simulink model "boundingbox"  (R2018a)
settings: Solver=VariableStepAuto  StartTime=0.0  StopTime=10.0  RelTol=1e-3
libraries: simulink x127
(part 3 of 4)

== system boundingbox/generate_proximity_sensor_readings/Subsystem1/distance_to_bounding_box/calculate_intersection 2 ==
  note: for two 2d vectors U=(Ux,Uy) V=(Vx,Vy)the crossproduct isU x V = Ux*Vy-Uy*Vx
  vertex_1 : Inport
  vertex_2 : Inport  Port=2
  "origin " : Inport  Port=3
  ray : Inport  Port=4
  AND : Logic  Inputs=3  IconShape=distinctive  AllPortsSameDT=off  OutDataTypeStr=boolean
  Abs : Abs
  Compare To Constant : simulink/Logic and Bit Operations/Compare To Constant  relop=<=  const=1  OutDataTypeStr=boolean
  Compare To Zero : simulink/Logic and Bit Operations/Compare To Zero  relop=>=  OutDataTypeStr=boolean
  Compare To Zero1 : simulink/Logic and Bit Operations/Compare To Zero  relop=>=  OutDataTypeStr=boolean
  Demux{,1..6} (7 alike) : Demux  Outputs=2
  Divide : Product  Inputs=*/
  Divide1 : Product  Inputs=*/
  Dot Product : DotProduct  InputSameDT=on  OutDataTypeStr=Inherit: Inherit via internal rule
  Dot Product1 : DotProduct  InputSameDT=on  OutDataTypeStr=Inherit: Inherit via internal rule
  Dot Product2 : DotProduct  InputSameDT=on  OutDataTypeStr=Inherit: Inherit via internal rule
  Gain : Gain  Gain=-1
  Multiply : Product
  Multiply1 : Product
  Subtract{,1,3..4} (4 alike) : Sum  Inputs=-+
  Subtract2 : Sum  Inputs=+-
  Vector Concatenate : Concatenate
  Vector Concatenate1 : Concatenate
  Vector Concatenate2 : Concatenate
  distance : Outport
  intersection (0,1) : Outport  Port=2
  wires:
  Compare To Constant/1 -> AND/3
  Compare To Zero/1 -> AND/2
  Divide1/1 -> Compare To Zero/1, Compare To Constant/1
  AND/1 -> intersection (0,1)/1
  Dot Product2/1 -> Divide1/2
  Dot Product1/1 -> Divide1/1
  Multiply1/1 -> Subtract2/2
  Multiply/1 -> Subtract2/1
  Demux2/1 -> Multiply1/2
  Demux1/2 -> Multiply1/1
  Demux2/2 -> Multiply/2
  Demux1/1 -> Multiply/1
  Abs/1 -> Divide/1
  Subtract2/1 -> Abs/1
  Dot Product/1 -> Divide/2
  Divide/1 -> Compare To Zero1/1, distance/1
  Subtract/1 -> Vector Concatenate1/2
  Vector Concatenate/1 -> Dot Product/2, Dot Product1/2, Dot Product2/2
  Demux/1 -> Vector Concatenate/2
  Gain/1 -> Vector Concatenate/1
  Demux/2 -> Gain/1
  ray/1 -> Demux/1
  vertex_2/1 -> Demux3/1
  vertex_1/1 -> Demux6/1, Demux4/1
  "origin "/1 -> Demux5/1
  Demux5/1 -> Subtract3/2
  Demux6/1 -> Subtract3/1
  Demux6/2 -> Subtract/1
  Demux5/2 -> Subtract/2
  Demux4/1 -> Subtract1/1
  Demux4/2 -> Subtract4/1
  Demux3/1 -> Subtract1/2
  Demux3/2 -> Subtract4/2
  Subtract3/1 -> Vector Concatenate1/1
  Vector Concatenate1/1 -> Dot Product1/1, Demux1/1
  Subtract4/1 -> Vector Concatenate2/2
  Subtract1/1 -> Vector Concatenate2/1
  Vector Concatenate2/1 -> Dot Product/1, Demux2/1, Dot Product2/1
  Compare To Zero1/1 -> AND/1

== system boundingbox/generate_proximity_sensor_readings/Subsystem1/distance_to_bounding_box/calculate_intersection 3 ==
  note: for two 2d vectors U=(Ux,Uy) V=(Vx,Vy)the crossproduct isU x V = Ux*Vy-Uy*Vx
  vertex_1 : Inport
  vertex_2 : Inport  Port=2
  "origin " : Inport  Port=3
  ray : Inport  Port=4
  AND : Logic  Inputs=3  IconShape=distinctive  AllPortsSameDT=off  OutDataTypeStr=boolean
  Abs : Abs
  Compare To Constant : simulink/Logic and Bit Operations/Compare To Constant  relop=<=  const=1  OutDataTypeStr=boolean
  Compare To Zero : simulink/Logic and Bit Operations/Compare To Zero  relop=>=  OutDataTypeStr=boolean
  Compare To Zero1 : simulink/Logic and Bit Operations/Compare To Zero  relop=>=  OutDataTypeStr=boolean
  Demux{,1..6} (7 alike) : Demux  Outputs=2
  Divide : Product  Inputs=*/
  Divide1 : Product  Inputs=*/
  Dot Product : DotProduct  InputSameDT=on  OutDataTypeStr=Inherit: Inherit via internal rule
  Dot Product1 : DotProduct  InputSameDT=on  OutDataTypeStr=Inherit: Inherit via internal rule
  Dot Product2 : DotProduct  InputSameDT=on  OutDataTypeStr=Inherit: Inherit via internal rule
  Gain : Gain  Gain=-1
  Multiply : Product
  Multiply1 : Product
  Subtract{,1,3..4} (4 alike) : Sum  Inputs=-+
  Subtract2 : Sum  Inputs=+-
  Vector Concatenate : Concatenate
  Vector Concatenate1 : Concatenate
  Vector Concatenate2 : Concatenate
  distance : Outport
  intersection (0,1) : Outport  Port=2
  wires:
  Compare To Zero1/1 -> AND/1
  Vector Concatenate2/1 -> Dot Product2/1, Demux2/1, Dot Product/1
  Subtract1/1 -> Vector Concatenate2/1
  Subtract4/1 -> Vector Concatenate2/2
  Vector Concatenate1/1 -> Demux1/1, Dot Product1/1
  Subtract3/1 -> Vector Concatenate1/1
  Demux3/2 -> Subtract4/2
  Demux3/1 -> Subtract1/2
  Demux4/2 -> Subtract4/1
  Demux4/1 -> Subtract1/1
  Demux5/2 -> Subtract/2
  Demux6/2 -> Subtract/1
  Demux6/1 -> Subtract3/1
  Demux5/1 -> Subtract3/2
  "origin "/1 -> Demux5/1
  vertex_1/1 -> Demux4/1, Demux6/1
  vertex_2/1 -> Demux3/1
  ray/1 -> Demux/1
  Demux/2 -> Gain/1
  Gain/1 -> Vector Concatenate/1
  Demux/1 -> Vector Concatenate/2
  Vector Concatenate/1 -> Dot Product2/2, Dot Product1/2, Dot Product/2
  Subtract/1 -> Vector Concatenate1/2
  Divide/1 -> distance/1, Compare To Zero1/1
  Dot Product/1 -> Divide/2
  Subtract2/1 -> Abs/1
  Abs/1 -> Divide/1
  Demux1/1 -> Multiply/1
  Demux2/2 -> Multiply/2
  Demux1/2 -> Multiply1/1
  Demux2/1 -> Multiply1/2
  Multiply/1 -> Subtract2/1
  Multiply1/1 -> Subtract2/2
  Dot Product1/1 -> Divide1/1
  Dot Product2/1 -> Divide1/2
  AND/1 -> intersection (0,1)/1
  Divide1/1 -> Compare To Constant/1, Compare To Zero/1
  Compare To Zero/1 -> AND/2
  Compare To Constant/1 -> AND/3

== system boundingbox/generate_proximity_sensor_readings/Subsystem1/distance_to_bounding_box1/calculate_intersection  ==
  note: for two 2d vectors U=(Ux,Uy) V=(Vx,Vy)the crossproduct isU x V = Ux*Vy-Uy*Vx
  vertex_1 : Inport
  vertex_2 : Inport  Port=2
  "origin " : Inport  Port=3
  ray : Inport  Port=4
  AND : Logic  Inputs=3  IconShape=distinctive  AllPortsSameDT=off  OutDataTypeStr=boolean
  Abs : Abs
  Compare To Constant : simulink/Logic and Bit Operations/Compare To Constant  relop=<=  const=1  OutDataTypeStr=boolean
  Compare To Zero : simulink/Logic and Bit Operations/Compare To Zero  relop=>=  OutDataTypeStr=boolean
  Compare To Zero1 : simulink/Logic and Bit Operations/Compare To Zero  relop=>=  OutDataTypeStr=boolean
  Demux{,1..6} (7 alike) : Demux  Outputs=2
  Divide : Product  Inputs=*/
  Divide1 : Product  Inputs=*/
  Dot Product : DotProduct  InputSameDT=on  OutDataTypeStr=Inherit: Inherit via internal rule
  Dot Product1 : DotProduct  InputSameDT=on  OutDataTypeStr=Inherit: Inherit via internal rule
  Dot Product2 : DotProduct  InputSameDT=on  OutDataTypeStr=Inherit: Inherit via internal rule
  Gain : Gain  Gain=-1
  Multiply : Product
  Multiply1 : Product
  Subtract{,1,3..4} (4 alike) : Sum  Inputs=-+
  Subtract2 : Sum  Inputs=+-
  Vector Concatenate : Concatenate
  Vector Concatenate1 : Concatenate
  Vector Concatenate2 : Concatenate
  distance : Outport
  intersection (0,1) : Outport  Port=2
  wires:
  Compare To Constant/1 -> AND/3
  Compare To Zero/1 -> AND/2
  Divide1/1 -> Compare To Zero/1, Compare To Constant/1
  AND/1 -> intersection (0,1)/1
  Dot Product2/1 -> Divide1/2
  Dot Product1/1 -> Divide1/1
  Multiply1/1 -> Subtract2/2
  Multiply/1 -> Subtract2/1
  Demux2/1 -> Multiply1/2
  Demux1/2 -> Multiply1/1
  Demux2/2 -> Multiply/2
  Demux1/1 -> Multiply/1
  Abs/1 -> Divide/1
  Subtract2/1 -> Abs/1
  Dot Product/1 -> Divide/2
  Divide/1 -> Compare To Zero1/1, distance/1
  Subtract/1 -> Vector Concatenate1/2
  Vector Concatenate/1 -> Dot Product/2, Dot Product1/2, Dot Product2/2
  Demux/1 -> Vector Concatenate/2
  Gain/1 -> Vector Concatenate/1
  Demux/2 -> Gain/1
  ray/1 -> Demux/1
  vertex_2/1 -> Demux3/1
  vertex_1/1 -> Demux6/1, Demux4/1
  "origin "/1 -> Demux5/1
  Demux5/1 -> Subtract3/2
  Demux6/1 -> Subtract3/1
  Demux6/2 -> Subtract/1
  Demux5/2 -> Subtract/2
  Demux4/1 -> Subtract1/1
  Demux4/2 -> Subtract4/1
  Demux3/1 -> Subtract1/2
  Demux3/2 -> Subtract4/2
  Subtract3/1 -> Vector Concatenate1/1
  Vector Concatenate1/1 -> Dot Product1/1, Demux1/1
  Subtract4/1 -> Vector Concatenate2/2
  Subtract1/1 -> Vector Concatenate2/1
  Vector Concatenate2/1 -> Dot Product/1, Demux2/1, Dot Product2/1
  Compare To Zero1/1 -> AND/1

== system boundingbox/generate_proximity_sensor_readings/Subsystem1/distance_to_bounding_box1/calculate_intersection 1 ==
  note: for two 2d vectors U=(Ux,Uy) V=(Vx,Vy)the crossproduct isU x V = Ux*Vy-Uy*Vx
  vertex_1 : Inport
  vertex_2 : Inport  Port=2
  "origin " : Inport  Port=3
  ray : Inport  Port=4
  AND : Logic  Inputs=3  IconShape=distinctive  AllPortsSameDT=off  OutDataTypeStr=boolean
  Abs : Abs
  Compare To Constant : simulink/Logic and Bit Operations/Compare To Constant  relop=<=  const=1  OutDataTypeStr=boolean
  Compare To Zero : simulink/Logic and Bit Operations/Compare To Zero  relop=>=  OutDataTypeStr=boolean
  Compare To Zero1 : simulink/Logic and Bit Operations/Compare To Zero  relop=>=  OutDataTypeStr=boolean
  Demux{,1..6} (7 alike) : Demux  Outputs=2
  Divide : Product  Inputs=*/
  Divide1 : Product  Inputs=*/
  Dot Product : DotProduct  InputSameDT=on  OutDataTypeStr=Inherit: Inherit via internal rule
  Dot Product1 : DotProduct  InputSameDT=on  OutDataTypeStr=Inherit: Inherit via internal rule
  Dot Product2 : DotProduct  InputSameDT=on  OutDataTypeStr=Inherit: Inherit via internal rule
  Gain : Gain  Gain=-1
  Multiply : Product
  Multiply1 : Product
  Subtract{,1,3..4} (4 alike) : Sum  Inputs=-+
  Subtract2 : Sum  Inputs=+-
  Vector Concatenate : Concatenate
  Vector Concatenate1 : Concatenate
  Vector Concatenate2 : Concatenate
  distance : Outport
  intersection (0,1) : Outport  Port=2
  wires:
  Compare To Zero1/1 -> AND/1
  Vector Concatenate2/1 -> Dot Product2/1, Demux2/1, Dot Product/1
  Subtract1/1 -> Vector Concatenate2/1
  Subtract4/1 -> Vector Concatenate2/2
  Vector Concatenate1/1 -> Demux1/1, Dot Product1/1
  Subtract3/1 -> Vector Concatenate1/1
  Demux3/2 -> Subtract4/2
  Demux3/1 -> Subtract1/2
  Demux4/2 -> Subtract4/1
  Demux4/1 -> Subtract1/1
  Demux5/2 -> Subtract/2
  Demux6/2 -> Subtract/1
  Demux6/1 -> Subtract3/1
  Demux5/1 -> Subtract3/2
  "origin "/1 -> Demux5/1
  vertex_1/1 -> Demux4/1, Demux6/1
  vertex_2/1 -> Demux3/1
  ray/1 -> Demux/1
  Demux/2 -> Gain/1
  Gain/1 -> Vector Concatenate/1
  Demux/1 -> Vector Concatenate/2
  Vector Concatenate/1 -> Dot Product2/2, Dot Product1/2, Dot Product/2
  Subtract/1 -> Vector Concatenate1/2
  Divide/1 -> distance/1, Compare To Zero1/1
  Dot Product/1 -> Divide/2
  Subtract2/1 -> Abs/1
  Abs/1 -> Divide/1
  Demux1/1 -> Multiply/1
  Demux2/2 -> Multiply/2
  Demux1/2 -> Multiply1/1
  Demux2/1 -> Multiply1/2
  Multiply/1 -> Subtract2/1
  Multiply1/1 -> Subtract2/2
  Dot Product1/1 -> Divide1/1
  Dot Product2/1 -> Divide1/2
  AND/1 -> intersection (0,1)/1
  Divide1/1 -> Compare To Constant/1, Compare To Zero/1
  Compare To Zero/1 -> AND/2
  Compare To Constant/1 -> AND/3

== system boundingbox/generate_proximity_sensor_readings/Subsystem1/distance_to_bounding_box1/calculate_intersection 2 ==
  note: for two 2d vectors U=(Ux,Uy) V=(Vx,Vy)the crossproduct isU x V = Ux*Vy-Uy*Vx
  vertex_1 : Inport
  vertex_2 : Inport  Port=2
  "origin " : Inport  Port=3
  ray : Inport  Port=4
  AND : Logic  Inputs=3  IconShape=distinctive  AllPortsSameDT=off  OutDataTypeStr=boolean
  Abs : Abs
  Compare To Constant : simulink/Logic and Bit Operations/Compare To Constant  relop=<=  const=1  OutDataTypeStr=boolean
  Compare To Zero : simulink/Logic and Bit Operations/Compare To Zero  relop=>=  OutDataTypeStr=boolean
  Compare To Zero1 : simulink/Logic and Bit Operations/Compare To Zero  relop=>=  OutDataTypeStr=boolean
  Demux{,1..6} (7 alike) : Demux  Outputs=2
  Divide : Product  Inputs=*/
  Divide1 : Product  Inputs=*/
  Dot Product : DotProduct  InputSameDT=on  OutDataTypeStr=Inherit: Inherit via internal rule
  Dot Product1 : DotProduct  InputSameDT=on  OutDataTypeStr=Inherit: Inherit via internal rule
  Dot Product2 : DotProduct  InputSameDT=on  OutDataTypeStr=Inherit: Inherit via internal rule
  Gain : Gain  Gain=-1
  Multiply : Product
  Multiply1 : Product
  Subtract{,1,3..4} (4 alike) : Sum  Inputs=-+
  Subtract2 : Sum  Inputs=+-
  Vector Concatenate : Concatenate
  Vector Concatenate1 : Concatenate
  Vector Concatenate2 : Concatenate
  distance : Outport
  intersection (0,1) : Outport  Port=2
  wires:
  Compare To Constant/1 -> AND/3
  Compare To Zero/1 -> AND/2
  Divide1/1 -> Compare To Zero/1, Compare To Constant/1
  AND/1 -> intersection (0,1)/1
  Dot Product2/1 -> Divide1/2
  Dot Product1/1 -> Divide1/1
  Multiply1/1 -> Subtract2/2
  Multiply/1 -> Subtract2/1
  Demux2/1 -> Multiply1/2
  Demux1/2 -> Multiply1/1
  Demux2/2 -> Multiply/2
  Demux1/1 -> Multiply/1
  Abs/1 -> Divide/1
  Subtract2/1 -> Abs/1
  Dot Product/1 -> Divide/2
  Divide/1 -> Compare To Zero1/1, distance/1
  Subtract/1 -> Vector Concatenate1/2
  Vector Concatenate/1 -> Dot Product/2, Dot Product1/2, Dot Product2/2
  Demux/1 -> Vector Concatenate/2
  Gain/1 -> Vector Concatenate/1
  Demux/2 -> Gain/1
  ray/1 -> Demux/1
  vertex_2/1 -> Demux3/1
  vertex_1/1 -> Demux6/1, Demux4/1
  "origin "/1 -> Demux5/1
  Demux5/1 -> Subtract3/2
  Demux6/1 -> Subtract3/1
  Demux6/2 -> Subtract/1
  Demux5/2 -> Subtract/2
  Demux4/1 -> Subtract1/1
  Demux4/2 -> Subtract4/1
  Demux3/1 -> Subtract1/2
  Demux3/2 -> Subtract4/2
  Subtract3/1 -> Vector Concatenate1/1
  Vector Concatenate1/1 -> Dot Product1/1, Demux1/1
  Subtract4/1 -> Vector Concatenate2/2
  Subtract1/1 -> Vector Concatenate2/1
  Vector Concatenate2/1 -> Dot Product/1, Demux2/1, Dot Product2/1
  Compare To Zero1/1 -> AND/1

== system boundingbox/generate_proximity_sensor_readings/Subsystem1/distance_to_bounding_box1/calculate_intersection 3 ==
  note: for two 2d vectors U=(Ux,Uy) V=(Vx,Vy)the crossproduct isU x V = Ux*Vy-Uy*Vx
  vertex_1 : Inport
  vertex_2 : Inport  Port=2
  "origin " : Inport  Port=3
  ray : Inport  Port=4
  AND : Logic  Inputs=3  IconShape=distinctive  AllPortsSameDT=off  OutDataTypeStr=boolean
  Abs : Abs
  Compare To Constant : simulink/Logic and Bit Operations/Compare To Constant  relop=<=  const=1  OutDataTypeStr=boolean
  Compare To Zero : simulink/Logic and Bit Operations/Compare To Zero  relop=>=  OutDataTypeStr=boolean
  Compare To Zero1 : simulink/Logic and Bit Operations/Compare To Zero  relop=>=  OutDataTypeStr=boolean
  Demux{,1..6} (7 alike) : Demux  Outputs=2
  Divide : Product  Inputs=*/
  Divide1 : Product  Inputs=*/
  Dot Product : DotProduct  InputSameDT=on  OutDataTypeStr=Inherit: Inherit via internal rule
  Dot Product1 : DotProduct  InputSameDT=on  OutDataTypeStr=Inherit: Inherit via internal rule
  Dot Product2 : DotProduct  InputSameDT=on  OutDataTypeStr=Inherit: Inherit via internal rule
  Gain : Gain  Gain=-1
  Multiply : Product
  Multiply1 : Product
  Subtract{,1,3..4} (4 alike) : Sum  Inputs=-+
  Subtract2 : Sum  Inputs=+-
  Vector Concatenate : Concatenate
  Vector Concatenate1 : Concatenate
  Vector Concatenate2 : Concatenate
  distance : Outport
  intersection (0,1) : Outport  Port=2
  wires:
  Compare To Zero1/1 -> AND/1
  Vector Concatenate2/1 -> Dot Product2/1, Demux2/1, Dot Product/1
  Subtract1/1 -> Vector Concatenate2/1
  Subtract4/1 -> Vector Concatenate2/2
  Vector Concatenate1/1 -> Demux1/1, Dot Product1/1
  Subtract3/1 -> Vector Concatenate1/1
  Demux3/2 -> Subtract4/2
  Demux3/1 -> Subtract1/2
  Demux4/2 -> Subtract4/1
  Demux4/1 -> Subtract1/1
  Demux5/2 -> Subtract/2
  Demux6/2 -> Subtract/1
  Demux6/1 -> Subtract3/1
  Demux5/1 -> Subtract3/2
  "origin "/1 -> Demux5/1
  vertex_1/1 -> Demux4/1, Demux6/1
  vertex_2/1 -> Demux3/1
  ray/1 -> Demux/1
  Demux/2 -> Gain/1
  Gain/1 -> Vector Concatenate/1
  Demux/1 -> Vector Concatenate/2
  Vector Concatenate/1 -> Dot Product2/2, Dot Product1/2, Dot Product/2
  Subtract/1 -> Vector Concatenate1/2
  Divide/1 -> distance/1, Compare To Zero1/1
  Dot Product/1 -> Divide/2
  Subtract2/1 -> Abs/1
  Abs/1 -> Divide/1
  Demux1/1 -> Multiply/1
  Demux2/2 -> Multiply/2
  Demux1/2 -> Multiply1/1
  Demux2/1 -> Multiply1/2
  Multiply/1 -> Subtract2/1
  Multiply1/1 -> Subtract2/2
  Dot Product1/1 -> Divide1/1
  Dot Product2/1 -> Divide1/2
  AND/1 -> intersection (0,1)/1
  Divide1/1 -> Compare To Constant/1, Compare To Zero/1
  Compare To Zero/1 -> AND/2
  Compare To Constant/1 -> AND/3

== system boundingbox/generate_proximity_sensor_readings/Subsystem1/distance_to_bounding_box2/calculate_intersection  ==
  note: for two 2d vectors U=(Ux,Uy) V=(Vx,Vy)the crossproduct isU x V = Ux*Vy-Uy*Vx
  vertex_1 : Inport
  vertex_2 : Inport  Port=2
  "origin " : Inport  Port=3
  ray : Inport  Port=4
  AND : Logic  Inputs=3  IconShape=distinctive  AllPortsSameDT=off  OutDataTypeStr=boolean
  Abs : Abs
  Compare To Constant : simulink/Logic and Bit Operations/Compare To Constant  relop=<=  const=1  OutDataTypeStr=boolean
  Compare To Zero : simulink/Logic and Bit Operations/Compare To Zero  relop=>=  OutDataTypeStr=boolean
  Compare To Zero1 : simulink/Logic and Bit Operations/Compare To Zero  relop=>=  OutDataTypeStr=boolean
  Demux{,1..6} (7 alike) : Demux  Outputs=2
  Divide : Product  Inputs=*/
  Divide1 : Product  Inputs=*/
  Dot Product : DotProduct  InputSameDT=on  OutDataTypeStr=Inherit: Inherit via internal rule
  Dot Product1 : DotProduct  InputSameDT=on  OutDataTypeStr=Inherit: Inherit via internal rule
  Dot Product2 : DotProduct  InputSameDT=on  OutDataTypeStr=Inherit: Inherit via internal rule
  Gain : Gain  Gain=-1
  Multiply : Product
  Multiply1 : Product
  Subtract{,1,3..4} (4 alike) : Sum  Inputs=-+
  Subtract2 : Sum  Inputs=+-
  Vector Concatenate : Concatenate
  Vector Concatenate1 : Concatenate
  Vector Concatenate2 : Concatenate
  distance : Outport
  intersection (0,1) : Outport  Port=2
  wires:
  Compare To Constant/1 -> AND/3
  Compare To Zero/1 -> AND/2
  Divide1/1 -> Compare To Zero/1, Compare To Constant/1
  AND/1 -> intersection (0,1)/1
  Dot Product2/1 -> Divide1/2
  Dot Product1/1 -> Divide1/1
  Multiply1/1 -> Subtract2/2
  Multiply/1 -> Subtract2/1
  Demux2/1 -> Multiply1/2
  Demux1/2 -> Multiply1/1
  Demux2/2 -> Multiply/2
  Demux1/1 -> Multiply/1
  Abs/1 -> Divide/1
  Subtract2/1 -> Abs/1
  Dot Product/1 -> Divide/2
  Divide/1 -> Compare To Zero1/1, distance/1
  Subtract/1 -> Vector Concatenate1/2
  Vector Concatenate/1 -> Dot Product/2, Dot Product1/2, Dot Product2/2
  Demux/1 -> Vector Concatenate/2
  Gain/1 -> Vector Concatenate/1
  Demux/2 -> Gain/1
  ray/1 -> Demux/1
  vertex_2/1 -> Demux3/1
  vertex_1/1 -> Demux6/1, Demux4/1
  "origin "/1 -> Demux5/1
  Demux5/1 -> Subtract3/2
  Demux6/1 -> Subtract3/1
  Demux6/2 -> Subtract/1
  Demux5/2 -> Subtract/2
  Demux4/1 -> Subtract1/1
  Demux4/2 -> Subtract4/1
  Demux3/1 -> Subtract1/2
  Demux3/2 -> Subtract4/2
  Subtract3/1 -> Vector Concatenate1/1
  Vector Concatenate1/1 -> Dot Product1/1, Demux1/1
  Subtract4/1 -> Vector Concatenate2/2
  Subtract1/1 -> Vector Concatenate2/1
  Vector Concatenate2/1 -> Dot Product/1, Demux2/1, Dot Product2/1
  Compare To Zero1/1 -> AND/1

== system boundingbox/generate_proximity_sensor_readings/Subsystem1/distance_to_bounding_box2/calculate_intersection 1 ==
  note: for two 2d vectors U=(Ux,Uy) V=(Vx,Vy)the crossproduct isU x V = Ux*Vy-Uy*Vx
  vertex_1 : Inport
  vertex_2 : Inport  Port=2
  "origin " : Inport  Port=3
  ray : Inport  Port=4
  AND : Logic  Inputs=3  IconShape=distinctive  AllPortsSameDT=off  OutDataTypeStr=boolean
  Abs : Abs
  Compare To Constant : simulink/Logic and Bit Operations/Compare To Constant  relop=<=  const=1  OutDataTypeStr=boolean
  Compare To Zero : simulink/Logic and Bit Operations/Compare To Zero  relop=>=  OutDataTypeStr=boolean
  Compare To Zero1 : simulink/Logic and Bit Operations/Compare To Zero  relop=>=  OutDataTypeStr=boolean
  Demux{,1..6} (7 alike) : Demux  Outputs=2
  Divide : Product  Inputs=*/
  Divide1 : Product  Inputs=*/
  Dot Product : DotProduct  InputSameDT=on  OutDataTypeStr=Inherit: Inherit via internal rule
  Dot Product1 : DotProduct  InputSameDT=on  OutDataTypeStr=Inherit: Inherit via internal rule
  Dot Product2 : DotProduct  InputSameDT=on  OutDataTypeStr=Inherit: Inherit via internal rule
  Gain : Gain  Gain=-1
  Multiply : Product
  Multiply1 : Product
  Subtract{,1,3..4} (4 alike) : Sum  Inputs=-+
  Subtract2 : Sum  Inputs=+-
  Vector Concatenate : Concatenate
  Vector Concatenate1 : Concatenate
  Vector Concatenate2 : Concatenate
  distance : Outport
  intersection (0,1) : Outport  Port=2
  wires:
  Compare To Zero1/1 -> AND/1
  Vector Concatenate2/1 -> Dot Product2/1, Demux2/1, Dot Product/1
  Subtract1/1 -> Vector Concatenate2/1
  Subtract4/1 -> Vector Concatenate2/2
  Vector Concatenate1/1 -> Demux1/1, Dot Product1/1
  Subtract3/1 -> Vector Concatenate1/1
  Demux3/2 -> Subtract4/2
  Demux3/1 -> Subtract1/2
  Demux4/2 -> Subtract4/1
  Demux4/1 -> Subtract1/1
  Demux5/2 -> Subtract/2
  Demux6/2 -> Subtract/1
  Demux6/1 -> Subtract3/1
  Demux5/1 -> Subtract3/2
  "origin "/1 -> Demux5/1
  vertex_1/1 -> Demux4/1, Demux6/1
  vertex_2/1 -> Demux3/1
  ray/1 -> Demux/1
  Demux/2 -> Gain/1
  Gain/1 -> Vector Concatenate/1
  Demux/1 -> Vector Concatenate/2
  Vector Concatenate/1 -> Dot Product2/2, Dot Product1/2, Dot Product/2
  Subtract/1 -> Vector Concatenate1/2
  Divide/1 -> distance/1, Compare To Zero1/1
  Dot Product/1 -> Divide/2
  Subtract2/1 -> Abs/1
  Abs/1 -> Divide/1
  Demux1/1 -> Multiply/1
  Demux2/2 -> Multiply/2
  Demux1/2 -> Multiply1/1
  Demux2/1 -> Multiply1/2
  Multiply/1 -> Subtract2/1
  Multiply1/1 -> Subtract2/2
  Dot Product1/1 -> Divide1/1
  Dot Product2/1 -> Divide1/2
  AND/1 -> intersection (0,1)/1
  Divide1/1 -> Compare To Constant/1, Compare To Zero/1
  Compare To Zero/1 -> AND/2
  Compare To Constant/1 -> AND/3

== system boundingbox/generate_proximity_sensor_readings/Subsystem1/distance_to_bounding_box2/calculate_intersection 2 ==
  note: for two 2d vectors U=(Ux,Uy) V=(Vx,Vy)the crossproduct isU x V = Ux*Vy-Uy*Vx
  vertex_1 : Inport
  vertex_2 : Inport  Port=2
  "origin " : Inport  Port=3
  ray : Inport  Port=4
  AND : Logic  Inputs=3  IconShape=distinctive  AllPortsSameDT=off  OutDataTypeStr=boolean
  Abs : Abs
  Compare To Constant : simulink/Logic and Bit Operations/Compare To Constant  relop=<=  const=1  OutDataTypeStr=boolean
  Compare To Zero : simulink/Logic and Bit Operations/Compare To Zero  relop=>=  OutDataTypeStr=boolean
  Compare To Zero1 : simulink/Logic and Bit Operations/Compare To Zero  relop=>=  OutDataTypeStr=boolean
  Demux{,1..6} (7 alike) : Demux  Outputs=2
  Divide : Product  Inputs=*/
  Divide1 : Product  Inputs=*/
  Dot Product : DotProduct  InputSameDT=on  OutDataTypeStr=Inherit: Inherit via internal rule
  Dot Product1 : DotProduct  InputSameDT=on  OutDataTypeStr=Inherit: Inherit via internal rule
  Dot Product2 : DotProduct  InputSameDT=on  OutDataTypeStr=Inherit: Inherit via internal rule
  Gain : Gain  Gain=-1
  Multiply : Product
  Multiply1 : Product
  Subtract{,1,3..4} (4 alike) : Sum  Inputs=-+
  Subtract2 : Sum  Inputs=+-
  Vector Concatenate : Concatenate
  Vector Concatenate1 : Concatenate
  Vector Concatenate2 : Concatenate
  distance : Outport
  intersection (0,1) : Outport  Port=2
  wires:
  Compare To Constant/1 -> AND/3
  Compare To Zero/1 -> AND/2
  Divide1/1 -> Compare To Zero/1, Compare To Constant/1
  AND/1 -> intersection (0,1)/1
  Dot Product2/1 -> Divide1/2
  Dot Product1/1 -> Divide1/1
  Multiply1/1 -> Subtract2/2
  Multiply/1 -> Subtract2/1
  Demux2/1 -> Multiply1/2
  Demux1/2 -> Multiply1/1
  Demux2/2 -> Multiply/2
  Demux1/1 -> Multiply/1
  Abs/1 -> Divide/1
  Subtract2/1 -> Abs/1
  Dot Product/1 -> Divide/2
  Divide/1 -> Compare To Zero1/1, distance/1
  Subtract/1 -> Vector Concatenate1/2
  Vector Concatenate/1 -> Dot Product/2, Dot Product1/2, Dot Product2/2
  Demux/1 -> Vector Concatenate/2
  Gain/1 -> Vector Concatenate/1
  Demux/2 -> Gain/1
  ray/1 -> Demux/1
  vertex_2/1 -> Demux3/1
  vertex_1/1 -> Demux6/1, Demux4/1
  "origin "/1 -> Demux5/1
  Demux5/1 -> Subtract3/2
  Demux6/1 -> Subtract3/1
  Demux6/2 -> Subtract/1
  Demux5/2 -> Subtract/2
  Demux4/1 -> Subtract1/1
  Demux4/2 -> Subtract4/1
  Demux3/1 -> Subtract1/2
  Demux3/2 -> Subtract4/2
  Subtract3/1 -> Vector Concatenate1/1
  Vector Concatenate1/1 -> Dot Product1/1, Demux1/1
  Subtract4/1 -> Vector Concatenate2/2
  Subtract1/1 -> Vector Concatenate2/1
  Vector Concatenate2/1 -> Dot Product/1, Demux2/1, Dot Product2/1
  Compare To Zero1/1 -> AND/1

== system boundingbox/generate_proximity_sensor_readings/Subsystem1/distance_to_bounding_box2/calculate_intersection 3 ==
  note: for two 2d vectors U=(Ux,Uy) V=(Vx,Vy)the crossproduct isU x V = Ux*Vy-Uy*Vx
  vertex_1 : Inport
  vertex_2 : Inport  Port=2
  "origin " : Inport  Port=3
  ray : Inport  Port=4
  AND : Logic  Inputs=3  IconShape=distinctive  AllPortsSameDT=off  OutDataTypeStr=boolean
  Abs : Abs
  Compare To Constant : simulink/Logic and Bit Operations/Compare To Constant  relop=<=  const=1  OutDataTypeStr=boolean
  Compare To Zero : simulink/Logic and Bit Operations/Compare To Zero  relop=>=  OutDataTypeStr=boolean
  Compare To Zero1 : simulink/Logic and Bit Operations/Compare To Zero  relop=>=  OutDataTypeStr=boolean
  Demux{,1..6} (7 alike) : Demux  Outputs=2
  Divide : Product  Inputs=*/
  Divide1 : Product  Inputs=*/
  Dot Product : DotProduct  InputSameDT=on  OutDataTypeStr=Inherit: Inherit via internal rule
  Dot Product1 : DotProduct  InputSameDT=on  OutDataTypeStr=Inherit: Inherit via internal rule
  Dot Product2 : DotProduct  InputSameDT=on  OutDataTypeStr=Inherit: Inherit via internal rule
  Gain : Gain  Gain=-1
  Multiply : Product
  Multiply1 : Product
  Subtract{,1,3..4} (4 alike) : Sum  Inputs=-+
  Subtract2 : Sum  Inputs=+-
  Vector Concatenate : Concatenate
  Vector Concatenate1 : Concatenate
  Vector Concatenate2 : Concatenate
  distance : Outport
  intersection (0,1) : Outport  Port=2
  wires:
  Compare To Zero1/1 -> AND/1
  Vector Concatenate2/1 -> Dot Product2/1, Demux2/1, Dot Product/1
  Subtract1/1 -> Vector Concatenate2/1
  Subtract4/1 -> Vector Concatenate2/2
  Vector Concatenate1/1 -> Demux1/1, Dot Product1/1
  Subtract3/1 -> Vector Concatenate1/1
  Demux3/2 -> Subtract4/2
  Demux3/1 -> Subtract1/2
  Demux4/2 -> Subtract4/1
  Demux4/1 -> Subtract1/1
  Demux5/2 -> Subtract/2
  Demux6/2 -> Subtract/1
  Demux6/1 -> Subtract3/1
  Demux5/1 -> Subtract3/2
  "origin "/1 -> Demux5/1
  vertex_1/1 -> Demux4/1, Demux6/1
  vertex_2/1 -> Demux3/1
  ray/1 -> Demux/1
  Demux/2 -> Gain/1
  Gain/1 -> Vector Concatenate/1
  Demux/1 -> Vector Concatenate/2
  Vector Concatenate/1 -> Dot Product2/2, Dot Product1/2, Dot Product/2
  Subtract/1 -> Vector Concatenate1/2
  Divide/1 -> distance/1, Compare To Zero1/1
  Dot Product/1 -> Divide/2
  Subtract2/1 -> Abs/1
  Abs/1 -> Divide/1
  Demux1/1 -> Multiply/1
  Demux2/2 -> Multiply/2
  Demux1/2 -> Multiply1/1
  Demux2/1 -> Multiply1/2
  Multiply/1 -> Subtract2/1
  Multiply1/1 -> Subtract2/2
  Dot Product1/1 -> Divide1/1
  Dot Product2/1 -> Divide1/2
  AND/1 -> intersection (0,1)/1
  Divide1/1 -> Compare To Constant/1, Compare To Zero/1
  Compare To Zero/1 -> AND/2
  Compare To Constant/1 -> AND/3

== system boundingbox/generate_proximity_sensor_readings/Subsystem2/distance_to_bounding_box/calculate_intersection  ==
  note: for two 2d vectors U=(Ux,Uy) V=(Vx,Vy)the crossproduct isU x V = Ux*Vy-Uy*Vx
  vertex_1 : Inport
  vertex_2 : Inport  Port=2
  "origin " : Inport  Port=3
  ray : Inport  Port=4
  AND : Logic  Inputs=3  IconShape=distinctive  AllPortsSameDT=off  OutDataTypeStr=boolean
  Abs : Abs
  Compare To Constant : simulink/Logic and Bit Operations/Compare To Constant  relop=<=  const=1  OutDataTypeStr=boolean
  Compare To Zero : simulink/Logic and Bit Operations/Compare To Zero  relop=>=  OutDataTypeStr=boolean
  Compare To Zero1 : simulink/Logic and Bit Operations/Compare To Zero  relop=>=  OutDataTypeStr=boolean
  Demux{,1..6} (7 alike) : Demux  Outputs=2
  Divide : Product  Inputs=*/
  Divide1 : Product  Inputs=*/
  Dot Product : DotProduct  InputSameDT=on  OutDataTypeStr=Inherit: Inherit via internal rule
  Dot Product1 : DotProduct  InputSameDT=on  OutDataTypeStr=Inherit: Inherit via internal rule
  Dot Product2 : DotProduct  InputSameDT=on  OutDataTypeStr=Inherit: Inherit via internal rule
  Gain : Gain  Gain=-1
  Multiply : Product
  Multiply1 : Product
  Subtract{,1,3..4} (4 alike) : Sum  Inputs=-+
  Subtract2 : Sum  Inputs=+-
  Vector Concatenate : Concatenate
  Vector Concatenate1 : Concatenate
  Vector Concatenate2 : Concatenate
  distance : Outport
  intersection (0,1) : Outport  Port=2
  wires:
  Compare To Constant/1 -> AND/3
  Compare To Zero/1 -> AND/2
  Divide1/1 -> Compare To Zero/1, Compare To Constant/1
  AND/1 -> intersection (0,1)/1
  Dot Product2/1 -> Divide1/2
  Dot Product1/1 -> Divide1/1
  Multiply1/1 -> Subtract2/2
  Multiply/1 -> Subtract2/1
  Demux2/1 -> Multiply1/2
  Demux1/2 -> Multiply1/1
  Demux2/2 -> Multiply/2
  Demux1/1 -> Multiply/1
  Abs/1 -> Divide/1
  Subtract2/1 -> Abs/1
  Dot Product/1 -> Divide/2
  Divide/1 -> Compare To Zero1/1, distance/1
  Subtract/1 -> Vector Concatenate1/2
  Vector Concatenate/1 -> Dot Product/2, Dot Product1/2, Dot Product2/2
  Demux/1 -> Vector Concatenate/2
  Gain/1 -> Vector Concatenate/1
  Demux/2 -> Gain/1
  ray/1 -> Demux/1
  vertex_2/1 -> Demux3/1
  vertex_1/1 -> Demux6/1, Demux4/1
  "origin "/1 -> Demux5/1
  Demux5/1 -> Subtract3/2
  Demux6/1 -> Subtract3/1
  Demux6/2 -> Subtract/1
  Demux5/2 -> Subtract/2
  Demux4/1 -> Subtract1/1
  Demux4/2 -> Subtract4/1
  Demux3/1 -> Subtract1/2
  Demux3/2 -> Subtract4/2
  Subtract3/1 -> Vector Concatenate1/1
  Vector Concatenate1/1 -> Dot Product1/1, Demux1/1
  Subtract4/1 -> Vector Concatenate2/2
  Subtract1/1 -> Vector Concatenate2/1
  Vector Concatenate2/1 -> Dot Product/1, Demux2/1, Dot Product2/1
  Compare To Zero1/1 -> AND/1

== system boundingbox/generate_proximity_sensor_readings/Subsystem2/distance_to_bounding_box/calculate_intersection 1 ==
  note: for two 2d vectors U=(Ux,Uy) V=(Vx,Vy)the crossproduct isU x V = Ux*Vy-Uy*Vx
  vertex_1 : Inport
  vertex_2 : Inport  Port=2
  "origin " : Inport  Port=3
  ray : Inport  Port=4
  AND : Logic  Inputs=3  IconShape=distinctive  AllPortsSameDT=off  OutDataTypeStr=boolean
  Abs : Abs
  Compare To Constant : simulink/Logic and Bit Operations/Compare To Constant  relop=<=  const=1  OutDataTypeStr=boolean
  Compare To Zero : simulink/Logic and Bit Operations/Compare To Zero  relop=>=  OutDataTypeStr=boolean
  Compare To Zero1 : simulink/Logic and Bit Operations/Compare To Zero  relop=>=  OutDataTypeStr=boolean
  Demux{,1..6} (7 alike) : Demux  Outputs=2
  Divide : Product  Inputs=*/
  Divide1 : Product  Inputs=*/
  Dot Product : DotProduct  InputSameDT=on  OutDataTypeStr=Inherit: Inherit via internal rule
  Dot Product1 : DotProduct  InputSameDT=on  OutDataTypeStr=Inherit: Inherit via internal rule
  Dot Product2 : DotProduct  InputSameDT=on  OutDataTypeStr=Inherit: Inherit via internal rule
  Gain : Gain  Gain=-1
  Multiply : Product
  Multiply1 : Product
  Subtract{,1,3..4} (4 alike) : Sum  Inputs=-+
  Subtract2 : Sum  Inputs=+-
  Vector Concatenate : Concatenate
  Vector Concatenate1 : Concatenate
  Vector Concatenate2 : Concatenate
  distance : Outport
  intersection (0,1) : Outport  Port=2
  wires:
  Compare To Zero1/1 -> AND/1
  Vector Concatenate2/1 -> Dot Product2/1, Demux2/1, Dot Product/1
  Subtract1/1 -> Vector Concatenate2/1
  Subtract4/1 -> Vector Concatenate2/2
  Vector Concatenate1/1 -> Demux1/1, Dot Product1/1
  Subtract3/1 -> Vector Concatenate1/1
  Demux3/2 -> Subtract4/2
  Demux3/1 -> Subtract1/2
  Demux4/2 -> Subtract4/1
  Demux4/1 -> Subtract1/1
  Demux5/2 -> Subtract/2
  Demux6/2 -> Subtract/1
  Demux6/1 -> Subtract3/1
  Demux5/1 -> Subtract3/2
  "origin "/1 -> Demux5/1
  vertex_1/1 -> Demux4/1, Demux6/1
  vertex_2/1 -> Demux3/1
  ray/1 -> Demux/1
  Demux/2 -> Gain/1
  Gain/1 -> Vector Concatenate/1
  Demux/1 -> Vector Concatenate/2
  Vector Concatenate/1 -> Dot Product2/2, Dot Product1/2, Dot Product/2
  Subtract/1 -> Vector Concatenate1/2
  Divide/1 -> distance/1, Compare To Zero1/1
  Dot Product/1 -> Divide/2
  Subtract2/1 -> Abs/1
  Abs/1 -> Divide/1
  Demux1/1 -> Multiply/1
  Demux2/2 -> Multiply/2
  Demux1/2 -> Multiply1/1
  Demux2/1 -> Multiply1/2
  Multiply/1 -> Subtract2/1
  Multiply1/1 -> Subtract2/2
  Dot Product1/1 -> Divide1/1
  Dot Product2/1 -> Divide1/2
  AND/1 -> intersection (0,1)/1
  Divide1/1 -> Compare To Constant/1, Compare To Zero/1
  Compare To Zero/1 -> AND/2
  Compare To Constant/1 -> AND/3

== system boundingbox/generate_proximity_sensor_readings/Subsystem2/distance_to_bounding_box/calculate_intersection 2 ==
  note: for two 2d vectors U=(Ux,Uy) V=(Vx,Vy)the crossproduct isU x V = Ux*Vy-Uy*Vx
  vertex_1 : Inport
  vertex_2 : Inport  Port=2
  "origin " : Inport  Port=3
  ray : Inport  Port=4
  AND : Logic  Inputs=3  IconShape=distinctive  AllPortsSameDT=off  OutDataTypeStr=boolean
  Abs : Abs
  Compare To Constant : simulink/Logic and Bit Operations/Compare To Constant  relop=<=  const=1  OutDataTypeStr=boolean
  Compare To Zero : simulink/Logic and Bit Operations/Compare To Zero  relop=>=  OutDataTypeStr=boolean
  Compare To Zero1 : simulink/Logic and Bit Operations/Compare To Zero  relop=>=  OutDataTypeStr=boolean
  Demux{,1..6} (7 alike) : Demux  Outputs=2
  Divide : Product  Inputs=*/
  Divide1 : Product  Inputs=*/
  Dot Product : DotProduct  InputSameDT=on  OutDataTypeStr=Inherit: Inherit via internal rule
  Dot Product1 : DotProduct  InputSameDT=on  OutDataTypeStr=Inherit: Inherit via internal rule
  Dot Product2 : DotProduct  InputSameDT=on  OutDataTypeStr=Inherit: Inherit via internal rule
  Gain : Gain  Gain=-1
  Multiply : Product
  Multiply1 : Product
  Subtract{,1,3..4} (4 alike) : Sum  Inputs=-+
  Subtract2 : Sum  Inputs=+-
  Vector Concatenate : Concatenate
  Vector Concatenate1 : Concatenate
  Vector Concatenate2 : Concatenate
  distance : Outport
  intersection (0,1) : Outport  Port=2
  wires:
  Compare To Constant/1 -> AND/3
  Compare To Zero/1 -> AND/2
  Divide1/1 -> Compare To Zero/1, Compare To Constant/1
  AND/1 -> intersection (0,1)/1
  Dot Product2/1 -> Divide1/2
  Dot Product1/1 -> Divide1/1
  Multiply1/1 -> Subtract2/2
  Multiply/1 -> Subtract2/1
  Demux2/1 -> Multiply1/2
  Demux1/2 -> Multiply1/1
  Demux2/2 -> Multiply/2
  Demux1/1 -> Multiply/1
  Abs/1 -> Divide/1
  Subtract2/1 -> Abs/1
  Dot Product/1 -> Divide/2
  Divide/1 -> Compare To Zero1/1, distance/1
  Subtract/1 -> Vector Concatenate1/2
  Vector Concatenate/1 -> Dot Product/2, Dot Product1/2, Dot Product2/2
  Demux/1 -> Vector Concatenate/2
  Gain/1 -> Vector Concatenate/1
  Demux/2 -> Gain/1
  ray/1 -> Demux/1
  vertex_2/1 -> Demux3/1
  vertex_1/1 -> Demux6/1, Demux4/1
  "origin "/1 -> Demux5/1
  Demux5/1 -> Subtract3/2
  Demux6/1 -> Subtract3/1
  Demux6/2 -> Subtract/1
  Demux5/2 -> Subtract/2
  Demux4/1 -> Subtract1/1
  Demux4/2 -> Subtract4/1
  Demux3/1 -> Subtract1/2
  Demux3/2 -> Subtract4/2
  Subtract3/1 -> Vector Concatenate1/1
  Vector Concatenate1/1 -> Dot Product1/1, Demux1/1
  Subtract4/1 -> Vector Concatenate2/2
  Subtract1/1 -> Vector Concatenate2/1
  Vector Concatenate2/1 -> Dot Product/1, Demux2/1, Dot Product2/1
  Compare To Zero1/1 -> AND/1

== system boundingbox/generate_proximity_sensor_readings/Subsystem2/distance_to_bounding_box/calculate_intersection 3 ==
  note: for two 2d vectors U=(Ux,Uy) V=(Vx,Vy)the crossproduct isU x V = Ux*Vy-Uy*Vx
  vertex_1 : Inport
  vertex_2 : Inport  Port=2
  "origin " : Inport  Port=3
  ray : Inport  Port=4
  AND : Logic  Inputs=3  IconShape=distinctive  AllPortsSameDT=off  OutDataTypeStr=boolean
  Abs : Abs
  Compare To Constant : simulink/Logic and Bit Operations/Compare To Constant  relop=<=  const=1  OutDataTypeStr=boolean
  Compare To Zero : simulink/Logic and Bit Operations/Compare To Zero  relop=>=  OutDataTypeStr=boolean
  Compare To Zero1 : simulink/Logic and Bit Operations/Compare To Zero  relop=>=  OutDataTypeStr=boolean
  Demux{,1..6} (7 alike) : Demux  Outputs=2
  Divide : Product  Inputs=*/
  Divide1 : Product  Inputs=*/
  Dot Product : DotProduct  InputSameDT=on  OutDataTypeStr=Inherit: Inherit via internal rule
  Dot Product1 : DotProduct  InputSameDT=on  OutDataTypeStr=Inherit: Inherit via internal rule
  Dot Product2 : DotProduct  InputSameDT=on  OutDataTypeStr=Inherit: Inherit via internal rule
  Gain : Gain  Gain=-1
  Multiply : Product
  Multiply1 : Product
  Subtract{,1,3..4} (4 alike) : Sum  Inputs=-+
  Subtract2 : Sum  Inputs=+-
  Vector Concatenate : Concatenate
  Vector Concatenate1 : Concatenate
  Vector Concatenate2 : Concatenate
  distance : Outport
  intersection (0,1) : Outport  Port=2
  wires:
  Compare To Zero1/1 -> AND/1
  Vector Concatenate2/1 -> Dot Product2/1, Demux2/1, Dot Product/1
  Subtract1/1 -> Vector Concatenate2/1
  Subtract4/1 -> Vector Concatenate2/2
  Vector Concatenate1/1 -> Demux1/1, Dot Product1/1
  Subtract3/1 -> Vector Concatenate1/1
  Demux3/2 -> Subtract4/2
  Demux3/1 -> Subtract1/2
  Demux4/2 -> Subtract4/1
  Demux4/1 -> Subtract1/1
  Demux5/2 -> Subtract/2
  Demux6/2 -> Subtract/1
  Demux6/1 -> Subtract3/1
  Demux5/1 -> Subtract3/2
  "origin "/1 -> Demux5/1
  vertex_1/1 -> Demux4/1, Demux6/1
  vertex_2/1 -> Demux3/1
  ray/1 -> Demux/1
  Demux/2 -> Gain/1
  Gain/1 -> Vector Concatenate/1
  Demux/1 -> Vector Concatenate/2
  Vector Concatenate/1 -> Dot Product2/2, Dot Product1/2, Dot Product/2
  Subtract/1 -> Vector Concatenate1/2
  Divide/1 -> distance/1, Compare To Zero1/1
  Dot Product/1 -> Divide/2
  Subtract2/1 -> Abs/1
  Abs/1 -> Divide/1
  Demux1/1 -> Multiply/1
  Demux2/2 -> Multiply/2
  Demux1/2 -> Multiply1/1
  Demux2/1 -> Multiply1/2
  Multiply/1 -> Subtract2/1
  Multiply1/1 -> Subtract2/2
  Dot Product1/1 -> Divide1/1
  Dot Product2/1 -> Divide1/2
  AND/1 -> intersection (0,1)/1
  Divide1/1 -> Compare To Constant/1, Compare To Zero/1
  Compare To Zero/1 -> AND/2
  Compare To Constant/1 -> AND/3

== system boundingbox/generate_proximity_sensor_readings/Subsystem2/distance_to_bounding_box1/calculate_intersection  ==
  note: for two 2d vectors U=(Ux,Uy) V=(Vx,Vy)the crossproduct isU x V = Ux*Vy-Uy*Vx
  vertex_1 : Inport
  vertex_2 : Inport  Port=2
  "origin " : Inport  Port=3
  ray : Inport  Port=4
  AND : Logic  Inputs=3  IconShape=distinctive  AllPortsSameDT=off  OutDataTypeStr=boolean
  Abs : Abs
  Compare To Constant : simulink/Logic and Bit Operations/Compare To Constant  relop=<=  const=1  OutDataTypeStr=boolean
  Compare To Zero : simulink/Logic and Bit Operations/Compare To Zero  relop=>=  OutDataTypeStr=boolean
  Compare To Zero1 : simulink/Logic and Bit Operations/Compare To Zero  relop=>=  OutDataTypeStr=boolean
  Demux{,1..6} (7 alike) : Demux  Outputs=2
  Divide : Product  Inputs=*/
  Divide1 : Product  Inputs=*/
  Dot Product : DotProduct  InputSameDT=on  OutDataTypeStr=Inherit: Inherit via internal rule
  Dot Product1 : DotProduct  InputSameDT=on  OutDataTypeStr=Inherit: Inherit via internal rule
  Dot Product2 : DotProduct  InputSameDT=on  OutDataTypeStr=Inherit: Inherit via internal rule
  Gain : Gain  Gain=-1
  Multiply : Product
  Multiply1 : Product
  Subtract{,1,3..4} (4 alike) : Sum  Inputs=-+
  Subtract2 : Sum  Inputs=+-
  Vector Concatenate : Concatenate
  Vector Concatenate1 : Concatenate
  Vector Concatenate2 : Concatenate
  distance : Outport
  intersection (0,1) : Outport  Port=2
  wires:
  Compare To Constant/1 -> AND/3
  Compare To Zero/1 -> AND/2
  Divide1/1 -> Compare To Zero/1, Compare To Constant/1
  AND/1 -> intersection (0,1)/1
  Dot Product2/1 -> Divide1/2
  Dot Product1/1 -> Divide1/1
  Multiply1/1 -> Subtract2/2
  Multiply/1 -> Subtract2/1
  Demux2/1 -> Multiply1/2
  Demux1/2 -> Multiply1/1
  Demux2/2 -> Multiply/2
  Demux1/1 -> Multiply/1
  Abs/1 -> Divide/1
  Subtract2/1 -> Abs/1
  Dot Product/1 -> Divide/2
  Divide/1 -> Compare To Zero1/1, distance/1
  Subtract/1 -> Vector Concatenate1/2
  Vector Concatenate/1 -> Dot Product/2, Dot Product1/2, Dot Product2/2
  Demux/1 -> Vector Concatenate/2
  Gain/1 -> Vector Concatenate/1
  Demux/2 -> Gain/1
  ray/1 -> Demux/1
  vertex_2/1 -> Demux3/1
  vertex_1/1 -> Demux6/1, Demux4/1
  "origin "/1 -> Demux5/1
  Demux5/1 -> Subtract3/2
  Demux6/1 -> Subtract3/1
  Demux6/2 -> Subtract/1
  Demux5/2 -> Subtract/2
  Demux4/1 -> Subtract1/1
  Demux4/2 -> Subtract4/1
  Demux3/1 -> Subtract1/2
  Demux3/2 -> Subtract4/2
  Subtract3/1 -> Vector Concatenate1/1
  Vector Concatenate1/1 -> Dot Product1/1, Demux1/1
  Subtract4/1 -> Vector Concatenate2/2
  Subtract1/1 -> Vector Concatenate2/1
  Vector Concatenate2/1 -> Dot Product/1, Demux2/1, Dot Product2/1
  Compare To Zero1/1 -> AND/1

== system boundingbox/generate_proximity_sensor_readings/Subsystem2/distance_to_bounding_box1/calculate_intersection 1 ==
  note: for two 2d vectors U=(Ux,Uy) V=(Vx,Vy)the crossproduct isU x V = Ux*Vy-Uy*Vx
  vertex_1 : Inport
  vertex_2 : Inport  Port=2
  "origin " : Inport  Port=3
  ray : Inport  Port=4
  AND : Logic  Inputs=3  IconShape=distinctive  AllPortsSameDT=off  OutDataTypeStr=boolean
  Abs : Abs
  Compare To Constant : simulink/Logic and Bit Operations/Compare To Constant  relop=<=  const=1  OutDataTypeStr=boolean
  Compare To Zero : simulink/Logic and Bit Operations/Compare To Zero  relop=>=  OutDataTypeStr=boolean
  Compare To Zero1 : simulink/Logic and Bit Operations/Compare To Zero  relop=>=  OutDataTypeStr=boolean
  Demux{,1..6} (7 alike) : Demux  Outputs=2
  Divide : Product  Inputs=*/
  Divide1 : Product  Inputs=*/
  Dot Product : DotProduct  InputSameDT=on  OutDataTypeStr=Inherit: Inherit via internal rule
  Dot Product1 : DotProduct  InputSameDT=on  OutDataTypeStr=Inherit: Inherit via internal rule
  Dot Product2 : DotProduct  InputSameDT=on  OutDataTypeStr=Inherit: Inherit via internal rule
  Gain : Gain  Gain=-1
  Multiply : Product
  Multiply1 : Product
  Subtract{,1,3..4} (4 alike) : Sum  Inputs=-+
  Subtract2 : Sum  Inputs=+-
  Vector Concatenate : Concatenate
  Vector Concatenate1 : Concatenate
  Vector Concatenate2 : Concatenate
  distance : Outport
  intersection (0,1) : Outport  Port=2
  wires:
  Compare To Zero1/1 -> AND/1
  Vector Concatenate2/1 -> Dot Product2/1, Demux2/1, Dot Product/1
  Subtract1/1 -> Vector Concatenate2/1
  Subtract4/1 -> Vector Concatenate2/2
  Vector Concatenate1/1 -> Demux1/1, Dot Product1/1
  Subtract3/1 -> Vector Concatenate1/1
  Demux3/2 -> Subtract4/2
  Demux3/1 -> Subtract1/2
  Demux4/2 -> Subtract4/1
  Demux4/1 -> Subtract1/1
  Demux5/2 -> Subtract/2
  Demux6/2 -> Subtract/1
  Demux6/1 -> Subtract3/1
  Demux5/1 -> Subtract3/2
  "origin "/1 -> Demux5/1
  vertex_1/1 -> Demux4/1, Demux6/1
  vertex_2/1 -> Demux3/1
  ray/1 -> Demux/1
  Demux/2 -> Gain/1
  Gain/1 -> Vector Concatenate/1
  Demux/1 -> Vector Concatenate/2
  Vector Concatenate/1 -> Dot Product2/2, Dot Product1/2, Dot Product/2
  Subtract/1 -> Vector Concatenate1/2
  Divide/1 -> distance/1, Compare To Zero1/1
  Dot Product/1 -> Divide/2
  Subtract2/1 -> Abs/1
  Abs/1 -> Divide/1
  Demux1/1 -> Multiply/1
  Demux2/2 -> Multiply/2
  Demux1/2 -> Multiply1/1
  Demux2/1 -> Multiply1/2
  Multiply/1 -> Subtract2/1
  Multiply1/1 -> Subtract2/2
  Dot Product1/1 -> Divide1/1
  Dot Product2/1 -> Divide1/2
  AND/1 -> intersection (0,1)/1
  Divide1/1 -> Compare To Constant/1, Compare To Zero/1
  Compare To Zero/1 -> AND/2
  Compare To Constant/1 -> AND/3

== system boundingbox/generate_proximity_sensor_readings/Subsystem2/distance_to_bounding_box1/calculate_intersection 2 ==
  note: for two 2d vectors U=(Ux,Uy) V=(Vx,Vy)the crossproduct isU x V = Ux*Vy-Uy*Vx
  vertex_1 : Inport
  vertex_2 : Inport  Port=2
  "origin " : Inport  Port=3
  ray : Inport  Port=4
  AND : Logic  Inputs=3  IconShape=distinctive  AllPortsSameDT=off  OutDataTypeStr=boolean
  Abs : Abs
  Compare To Constant : simulink/Logic and Bit Operations/Compare To Constant  relop=<=  const=1  OutDataTypeStr=boolean
  Compare To Zero : simulink/Logic and Bit Operations/Compare To Zero  relop=>=  OutDataTypeStr=boolean
  Compare To Zero1 : simulink/Logic and Bit Operations/Compare To Zero  relop=>=  OutDataTypeStr=boolean
  Demux{,1..6} (7 alike) : Demux  Outputs=2
  Divide : Product  Inputs=*/
  Divide1 : Product  Inputs=*/
  Dot Product : DotProduct  InputSameDT=on  OutDataTypeStr=Inherit: Inherit via internal rule
  Dot Product1 : DotProduct  InputSameDT=on  OutDataTypeStr=Inherit: Inherit via internal rule
  Dot Product2 : DotProduct  InputSameDT=on  OutDataTypeStr=Inherit: Inherit via internal rule
  Gain : Gain  Gain=-1
  Multiply : Product
  Multiply1 : Product
  Subtract{,1,3..4} (4 alike) : Sum  Inputs=-+
  Subtract2 : Sum  Inputs=+-
  Vector Concatenate : Concatenate
  Vector Concatenate1 : Concatenate
  Vector Concatenate2 : Concatenate
  distance : Outport
  intersection (0,1) : Outport  Port=2
  wires:
  Compare To Constant/1 -> AND/3
  Compare To Zero/1 -> AND/2
  Divide1/1 -> Compare To Zero/1, Compare To Constant/1
  AND/1 -> intersection (0,1)/1
  Dot Product2/1 -> Divide1/2
  Dot Product1/1 -> Divide1/1
  Multiply1/1 -> Subtract2/2
  Multiply/1 -> Subtract2/1
  Demux2/1 -> Multiply1/2
  Demux1/2 -> Multiply1/1
  Demux2/2 -> Multiply/2
  Demux1/1 -> Multiply/1
  Abs/1 -> Divide/1
  Subtract2/1 -> Abs/1
  Dot Product/1 -> Divide/2
  Divide/1 -> Compare To Zero1/1, distance/1
  Subtract/1 -> Vector Concatenate1/2
  Vector Concatenate/1 -> Dot Product/2, Dot Product1/2, Dot Product2/2
  Demux/1 -> Vector Concatenate/2
  Gain/1 -> Vector Concatenate/1
  Demux/2 -> Gain/1
  ray/1 -> Demux/1
  vertex_2/1 -> Demux3/1
  vertex_1/1 -> Demux6/1, Demux4/1
  "origin "/1 -> Demux5/1
  Demux5/1 -> Subtract3/2
  Demux6/1 -> Subtract3/1
  Demux6/2 -> Subtract/1
  Demux5/2 -> Subtract/2
  Demux4/1 -> Subtract1/1
  Demux4/2 -> Subtract4/1
  Demux3/1 -> Subtract1/2
  Demux3/2 -> Subtract4/2
  Subtract3/1 -> Vector Concatenate1/1
  Vector Concatenate1/1 -> Dot Product1/1, Demux1/1
  Subtract4/1 -> Vector Concatenate2/2
  Subtract1/1 -> Vector Concatenate2/1
  Vector Concatenate2/1 -> Dot Product/1, Demux2/1, Dot Product2/1
  Compare To Zero1/1 -> AND/1

== system boundingbox/generate_proximity_sensor_readings/Subsystem2/distance_to_bounding_box1/calculate_intersection 3 ==
  note: for two 2d vectors U=(Ux,Uy) V=(Vx,Vy)the crossproduct isU x V = Ux*Vy-Uy*Vx
  vertex_1 : Inport
  vertex_2 : Inport  Port=2
  "origin " : Inport  Port=3
  ray : Inport  Port=4
  AND : Logic  Inputs=3  IconShape=distinctive  AllPortsSameDT=off  OutDataTypeStr=boolean
  Abs : Abs
  Compare To Constant : simulink/Logic and Bit Operations/Compare To Constant  relop=<=  const=1  OutDataTypeStr=boolean
  Compare To Zero : simulink/Logic and Bit Operations/Compare To Zero  relop=>=  OutDataTypeStr=boolean
  Compare To Zero1 : simulink/Logic and Bit Operations/Compare To Zero  relop=>=  OutDataTypeStr=boolean
  Demux{,1..6} (7 alike) : Demux  Outputs=2
  Divide : Product  Inputs=*/
  Divide1 : Product  Inputs=*/
  Dot Product : DotProduct  InputSameDT=on  OutDataTypeStr=Inherit: Inherit via internal rule
  Dot Product1 : DotProduct  InputSameDT=on  OutDataTypeStr=Inherit: Inherit via internal rule
  Dot Product2 : DotProduct  InputSameDT=on  OutDataTypeStr=Inherit: Inherit via internal rule
  Gain : Gain  Gain=-1
  Multiply : Product
  Multiply1 : Product
  Subtract{,1,3..4} (4 alike) : Sum  Inputs=-+
  Subtract2 : Sum  Inputs=+-
  Vector Concatenate : Concatenate
  Vector Concatenate1 : Concatenate
  Vector Concatenate2 : Concatenate
  distance : Outport
  intersection (0,1) : Outport  Port=2
  wires:
  Compare To Zero1/1 -> AND/1
  Vector Concatenate2/1 -> Dot Product2/1, Demux2/1, Dot Product/1
  Subtract1/1 -> Vector Concatenate2/1
  Subtract4/1 -> Vector Concatenate2/2
  Vector Concatenate1/1 -> Demux1/1, Dot Product1/1
  Subtract3/1 -> Vector Concatenate1/1
  Demux3/2 -> Subtract4/2
  Demux3/1 -> Subtract1/2
  Demux4/2 -> Subtract4/1
  Demux4/1 -> Subtract1/1
  Demux5/2 -> Subtract/2
  Demux6/2 -> Subtract/1
  Demux6/1 -> Subtract3/1
  Demux5/1 -> Subtract3/2
  "origin "/1 -> Demux5/1
  vertex_1/1 -> Demux4/1, Demux6/1
  vertex_2/1 -> Demux3/1
  ray/1 -> Demux/1
  Demux/2 -> Gain/1
  Gain/1 -> Vector Concatenate/1
  Demux/1 -> Vector Concatenate/2
  Vector Concatenate/1 -> Dot Product2/2, Dot Product1/2, Dot Product/2
  Subtract/1 -> Vector Concatenate1/2
  Divide/1 -> distance/1, Compare To Zero1/1
  Dot Product/1 -> Divide/2
  Subtract2/1 -> Abs/1
  Abs/1 -> Divide/1
  Demux1/1 -> Multiply/1
  Demux2/2 -> Multiply/2
  Demux1/2 -> Multiply1/1
  Demux2/1 -> Multiply1/2
  Multiply/1 -> Subtract2/1
  Multiply1/1 -> Subtract2/2
  Dot Product1/1 -> Divide1/1
  Dot Product2/1 -> Divide1/2
  AND/1 -> intersection (0,1)/1
  Divide1/1 -> Compare To Constant/1, Compare To Zero/1
  Compare To Zero/1 -> AND/2
  Compare To Constant/1 -> AND/3

== system boundingbox/generate_proximity_sensor_readings/Subsystem2/distance_to_bounding_box2/calculate_intersection  ==
  note: for two 2d vectors U=(Ux,Uy) V=(Vx,Vy)the crossproduct isU x V = Ux*Vy-Uy*Vx
  vertex_1 : Inport
  vertex_2 : Inport  Port=2
  "origin " : Inport  Port=3
  ray : Inport  Port=4
  AND : Logic  Inputs=3  IconShape=distinctive  AllPortsSameDT=off  OutDataTypeStr=boolean
  Abs : Abs
  Compare To Constant : simulink/Logic and Bit Operations/Compare To Constant  relop=<=  const=1  OutDataTypeStr=boolean
  Compare To Zero : simulink/Logic and Bit Operations/Compare To Zero  relop=>=  OutDataTypeStr=boolean
  Compare To Zero1 : simulink/Logic and Bit Operations/Compare To Zero  relop=>=  OutDataTypeStr=boolean
  Demux{,1..6} (7 alike) : Demux  Outputs=2
  Divide : Product  Inputs=*/
  Divide1 : Product  Inputs=*/
  Dot Product : DotProduct  InputSameDT=on  OutDataTypeStr=Inherit: Inherit via internal rule
  Dot Product1 : DotProduct  InputSameDT=on  OutDataTypeStr=Inherit: Inherit via internal rule
  Dot Product2 : DotProduct  InputSameDT=on  OutDataTypeStr=Inherit: Inherit via internal rule
  Gain : Gain  Gain=-1
  Multiply : Product
  Multiply1 : Product
  Subtract{,1,3..4} (4 alike) : Sum  Inputs=-+
  Subtract2 : Sum  Inputs=+-
  Vector Concatenate : Concatenate
  Vector Concatenate1 : Concatenate
  Vector Concatenate2 : Concatenate
  distance : Outport
  intersection (0,1) : Outport  Port=2
  wires:
  Compare To Constant/1 -> AND/3
  Compare To Zero/1 -> AND/2
  Divide1/1 -> Compare To Zero/1, Compare To Constant/1
  AND/1 -> intersection (0,1)/1
  Dot Product2/1 -> Divide1/2
  Dot Product1/1 -> Divide1/1
  Multiply1/1 -> Subtract2/2
  Multiply/1 -> Subtract2/1
  Demux2/1 -> Multiply1/2
  Demux1/2 -> Multiply1/1
  Demux2/2 -> Multiply/2
  Demux1/1 -> Multiply/1
  Abs/1 -> Divide/1
  Subtract2/1 -> Abs/1
  Dot Product/1 -> Divide/2
  Divide/1 -> Compare To Zero1/1, distance/1
  Subtract/1 -> Vector Concatenate1/2
  Vector Concatenate/1 -> Dot Product/2, Dot Product1/2, Dot Product2/2
  Demux/1 -> Vector Concatenate/2
  Gain/1 -> Vector Concatenate/1
  Demux/2 -> Gain/1
  ray/1 -> Demux/1
  vertex_2/1 -> Demux3/1
  vertex_1/1 -> Demux6/1, Demux4/1
  "origin "/1 -> Demux5/1
  Demux5/1 -> Subtract3/2
  Demux6/1 -> Subtract3/1
  Demux6/2 -> Subtract/1
  Demux5/2 -> Subtract/2
  Demux4/1 -> Subtract1/1
  Demux4/2 -> Subtract4/1
  Demux3/1 -> Subtract1/2
  Demux3/2 -> Subtract4/2
  Subtract3/1 -> Vector Concatenate1/1
  Vector Concatenate1/1 -> Dot Product1/1, Demux1/1
  Subtract4/1 -> Vector Concatenate2/2
  Subtract1/1 -> Vector Concatenate2/1
  Vector Concatenate2/1 -> Dot Product/1, Demux2/1, Dot Product2/1
  Compare To Zero1/1 -> AND/1
